simulink model "CRC"  (R2013a)
settings: Solver=ode45  StartTime=0.0  StopTime=10.0  RelTol=1e-3
undefined symbols (not defined in the file or in its folder): CRC, get
libraries: commcrc2 x2, dspsnks4 x2, commrandsrc2 x1, commchan3 x1, commsink2 x1
settings Model: Creator=sliencer  LastModifiedBy=sliencer

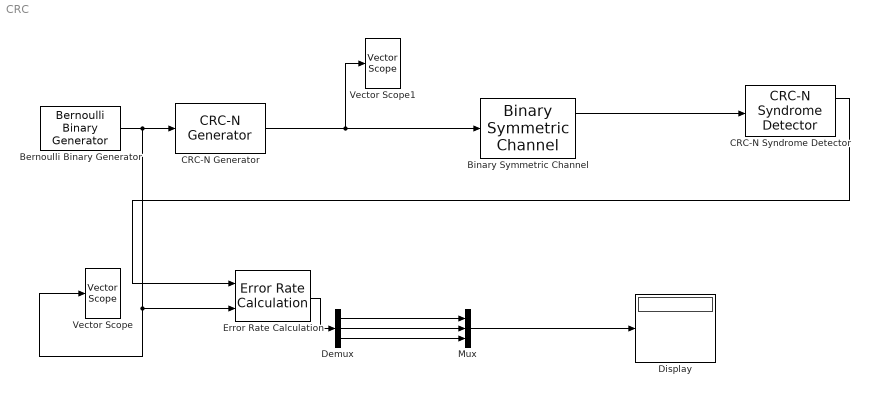
== system CRC ==
  Bernoulli Binary Generator : commrandsrc2/Bernoulli Binary Generator  P=0.5  seed=100  Ts=1  frameBased=on  sampPerFrame=20  orient=off  outDataType=double
  Binary Symmetric Channel : commchan3/Binary Symmetric Channel  P=0.1  s=71  E=on  outDtype=double
  CRC-N Generator : commcrc2/CRC-N Generator  crcMethod=CRC-16  iniStates=[0]  numChecksums=1
  CRC-N Syndrome Detector : commcrc2/CRC-N Syndrome Detector  crcMethod=CRC-16  iniStates=[0]  numChecksums=1
  Demux : Demux  Outputs=3
  Display : Display
      settings: Decimation=3
  Error Rate Calculation : commsink2/Error Rate Calculation  N=0  st_delay=0  cp_mode=Entire frame  subframe=[]  PMode=Port  WsName=ErrorVec  RsMode2=off  stop=off  numErr=100  maxBits=1e6
  Mux : Mux  Inputs=3
  Vector Scope : dspsnks4/Vector Scope  ScopeProperties=on  Domain=Time  HorizSpan=1  DisplayProperties=off  AxisGrid=on  Memory=off  FrameNumber=on  AxisLegend=off  AxisZoom=off  OpenScopeAtSimStart=on  OpenScopeImmediately=off  FigPos=get(0,'defaultfigureposition')  AxisProperties=off  XUnits=Hertz  XRange=[0...Fs/2]  InheritXIncr=on  XIncr=1  XLabel=Time  XLimit=Auto  XMin=0  XMax=1  XStart=0  YUnits=dB  YLabel=Amplitude  LineProperties=off  LineStyles=-  LineMarkers=*  XAxisParamsVer=6.9
      settings: YMin=-10  YMax=10
  Vector Scope1 : dspsnks4/Vector Scope  ScopeProperties=on  Domain=Time  HorizSpan=1  DisplayProperties=off  AxisGrid=on  Memory=off  FrameNumber=on  AxisLegend=off  AxisZoom=off  OpenScopeAtSimStart=on  OpenScopeImmediately=off  FigPos=get(0,'defaultfigureposition')  AxisProperties=off  XUnits=Hertz  XRange=[0...Fs/2]  InheritXIncr=on  XIncr=1  XLabel=Time  XLimit=Auto  XMin=0  XMax=1  XStart=0  YUnits=dB  YLabel=Amplitude  LineProperties=off  LineStyles=-  LineMarkers=*  XAxisParamsVer=6.9
      settings: YMin=-10  YMax=10
  wires:
  Bernoulli Binary Generator/1 -> Vector Scope/1, Error Rate Calculation/2, CRC-N Generator/1
  CRC-N Generator/1 -> Vector Scope1/1, Binary Symmetric Channel/1
  Binary Symmetric Channel/1 -> CRC-N Syndrome Detector/1
  CRC-N Syndrome Detector/1 -> Error Rate Calculation/1
  Demux/1 -> Mux/1
  Demux/2 -> Mux/2
  Demux/3 -> Mux/3
  Mux/1 -> Display/1
  Error Rate Calculation/1 -> Demux/1
